simulink model "PhysicalArchitecture"  (R2020b)
settings: Solver=VariableStepAuto  StartTime=0.0  StopTime=10.0  RelTol=1e-3
model workspace (MAT data in the model file):
  DataToReport = Simulink.Bus
  DataToReport.Alignment = -1
  DataToReport.Elements_internal(1) = Simulink.BusElement
  DataToReport.Elements_internal(1).DimensionsMode = 'Fixed'
  DataToReport.Elements_internal(1).SamplingMode = 'Sample based'
  DataToReport.Elements_internal(1).SampleTime = -1
  DataToReport.Elements_internal(1).Name = 'Waypoints'
  DataToReport.Elements_internal(1).DataType_internal = 'double'
  DataToReport.Elements_internal(1).Complexity = 'real'
  DataToReport.Elements_internal(1).Dimensions = 1
  DataToReport.Elements_internal(2) = Simulink.BusElement
  DataToReport.Elements_internal(2).DimensionsMode = 'Fixed'
  DataToReport.Elements_internal(2).SamplingMode = 'Sample based'
  DataToReport.Elements_internal(2).SampleTime = -1
  DataToReport.Elements_internal(2).Name = 'VehicleLocation'
  DataToReport.Elements_internal(2).DataType_internal = 'double'
  DataToReport.Elements_internal(2).Complexity = 'real'
  DataToReport.Elements_internal(2).Dimensions = 1
  DataToReport.Elements_internal(3) = Simulink.BusElement
  DataToReport.Elements_internal(3).DimensionsMode = 'Fixed'
  DataToReport.Elements_internal(3).SamplingMode = 'Sample based'
  DataToReport.Elements_internal(3).SampleTime = -1
  DataToReport.Elements_internal(3).Name = 'TargetLocation'
  DataToReport.Elements_internal(3).DataType_internal = 'double'
  DataToReport.Elements_internal(3).Complexity = 'real'
  DataToReport.Elements_internal(3).Dimensions = 1
  DataToReport.Elements_internal(4) = Simulink.BusElement
  DataToReport.Elements_internal(4).DimensionsMode = 'Fixed'
  DataToReport.Elements_internal(4).SamplingMode = 'Sample based'
  DataToReport.Elements_internal(4).SampleTime = -1
  DataToReport.Elements_internal(4).Name = 'BatteryLevel'
  DataToReport.Elements_internal(4).DataType_internal = 'double'
  DataToReport.Elements_internal(4).Complexity = 'real'
  DataToReport.Elements_internal(4).Dimensions = 1
  DataToReport.DataScope = 'Auto'
settings Model: OrderedModelArguments=off  Creator=jantonio  LastModifiedBy=jantonio

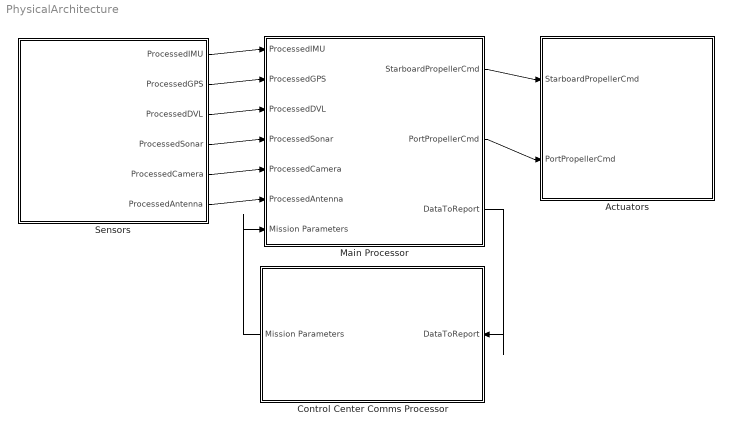
== system PhysicalArchitecture ==
  Actuators : Subsystem
      settings: PortSchema="{\"entries\":[{\"content\":{\"headerSize\":26,\"margin\":15,\"minimumSpacing\":25,\"sides\":[{\"content\":{\"connectorIds\":[\"In1\",\"In2\"]},\"type\":\"ConnectorPlacement.EquallySpacedRectSide\",\"uuid\":\"92d6a8cb-947e-47d6-81f8-e687db23cc48\"},{\"content\":{\"connectorIds\":[],\"side\":\"RIGHT\"},\"type\":\"ConnectorPlacement.EquallySpacedRectSide\",\"uuid\":\"2f71feb6-2a58-4436-853a-8f489ba40545\"},{\"content\":{\"connectorIds\":[],\"side\":\"TOP\"},\"type\":\"ConnectorPlacement.EquallySpacedRectSide\",\"uuid\":\"53be6a6a-df16-4e38-99d9-cb729dcfb7aa\"}]},\"type\":\"ConnectorPlacement.EquallySpacedConnector\",\"uuid\":\"6f13b966-c9d6-4990-a53d-58e940ab2e2e\"}],\"packageUris\":[\"http://schema.mathworks.com/mf0/Connector/19700101\"],\"version\":\"1.0\"}"
  Control Center Comms Processor : Subsystem
      settings: PortSchema="{\"entries\":[{\"content\":{\"headerSize\":26,\"margin\":15,\"minimumSpacing\":25,\"sides\":[{\"content\":{\"connectorIds\":[\"Out1\"]},\"type\":\"ConnectorPlacement.EquallySpacedRectSide\",\"uuid\":\"92d6a8cb-947e-47d6-81f8-e687db23cc48\"},{\"content\":{\"connectorIds\":[\"In1\"],\"side\":\"RIGHT\"},\"type\":\"ConnectorPlacement.EquallySpacedRectSide\",\"uuid\":\"2f71feb6-2a58-4436-853a-8f489ba40545\"},{\"content\":{\"connectorIds\":[],\"side\":\"TOP\"},\"type\":\"ConnectorPlacement.EquallySpacedRectSide\",\"uuid\":\"53be6a6a-df16-4e38-99d9-cb729dcfb7aa\"}]},\"type\":\"ConnectorPlacement.EquallySpacedConnector\",\"uuid\":\"6f13b966-c9d6-4990-a53d-58e940ab2e2e\"}],\"packageUris\":[\"http://schema.mathworks.com/mf0/Connector/19700101\"],\"version\":\"1.0\"}"
  Main Processor : Subsystem
      settings: PortSchema="{\"entries\":[{\"content\":{\"headerSize\":26,\"margin\":15,\"minimumSpacing\":25,\"sides\":[{\"content\":{\"connectorIds\":[\"In3\",\"In2\",\"In4\",\"In5\",\"In6\",\"In7\",\"In1\"]},\"type\":\"ConnectorPlacement.EquallySpacedRectSide\",\"uuid\":\"92d6a8cb-947e-47d6-81f8-e687db23cc48\"},{\"content\":{\"connectorIds\":[\"Out1\",\"Out2\",\"Out3\"],\"side\":\"RIGHT\"},\"type\":\"ConnectorPlacement.EquallySpacedRectSide\",\"uuid\":\"2f71feb6-2a58-4436-853a-8f489ba40545\"},{\"content\":{\"connectorIds\":[],\"side\":\"TOP\"},\"type\":\"ConnectorPlacement.EquallySpacedRectSide\",\"uuid\":\"53be6a6a-df16-4e38-99d9-cb729dcfb7aa\"},{\"content\":{\"connectorIds\":[],\"side\":\"BOTTOM\"},\"type\":\"ConnectorPlacement.EquallySpacedRectSide\",\"uuid\":\"d53c4466-3fe3-4f56-83bf-6f2fb5a5afe1\"}]},\"type\":\"ConnectorPlacement.EquallySpacedConnector\",\"uuid\":\"6f13b966-c9d6-4990-a53d-58e940ab2e2e\"}],\"packageUris\":[\"http://schema.mathworks.com/mf0/Connector/19700101\"],\"version\":\"1.0\"}"
  Sensors : Subsystem
      settings: PortSchema="{\"entries\":[{\"content\":{\"headerSize\":26,\"margin\":15,\"minimumSpacing\":25,\"sides\":[{\"content\":{\"connectorIds\":[]},\"type\":\"ConnectorPlacement.EquallySpacedRectSide\",\"uuid\":\"ebeba1ac-198c-4738-ae02-dee736f3e255\"},{\"content\":{\"connectorIds\":[\"Out1\",\"Out2\",\"Out3\",\"Out4\",\"Out6\",\"Out5\"],\"side\":\"RIGHT\"},\"type\":\"ConnectorPlacement.EquallySpacedRectSide\",\"uuid\":\"9a9b5092-10f1-44a7-a087-51aace0dbe34\"},{\"content\":{\"connectorIds\":[],\"side\":\"TOP\"},\"type\":\"ConnectorPlacement.EquallySpacedRectSide\",\"uuid\":\"96b74760-e30f-4e99-a3da-f77ce842a435\"}]},\"type\":\"ConnectorPlacement.EquallySpacedConnector\",\"uuid\":\"07af2d66-a99a-41b4-9a6d-4df096fe3f6b\"}],\"packageUris\":[\"http://schema.mathworks.com/mf0/Connector/19700101\"],\"version\":\"1.0\"}"
  wires:
  Sensors/1(ProcessedIMU) -> Main Processor/3(ProcessedIMU)
  Sensors/2(ProcessedGPS) -> Main Processor/2(ProcessedGPS)
  Sensors/5(ProcessedAntenna) -> Main Processor/7(ProcessedAntenna)
  Sensors/6(ProcessedCamera) -> Main Processor/6(ProcessedCamera)
  Sensors/4(ProcessedSonar) -> Main Processor/5(ProcessedSonar)
  Sensors/3(ProcessedDVL) -> Main Processor/4(ProcessedDVL)
  Main Processor/1(StarboardPropellerCmd) -> Actuators/1(StarboardPropellerCmd)
  Main Processor/2(PortPropellerCmd) -> Actuators/2(PortPropellerCmd)
  Control Center Comms Processor/1(Mission Parameters) -> Main Processor/1(Mission Parameters)
  Main Processor/3(DataToReport) -> Control Center Comms Processor/1(DataToReport)

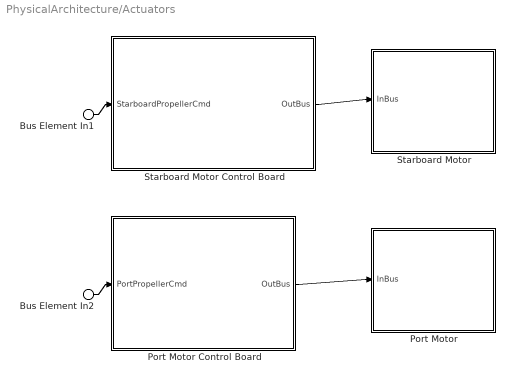
== system PhysicalArchitecture/Actuators ==
  Bus Element In1 : Inport  PortName=StarboardPropellerCmd
  Bus Element In2 : Inport  Port=2  PortName=PortPropellerCmd
  Port Motor : Subsystem
      settings: PortSchema="{\"entries\":[{\"content\":{\"headerSize\":26,\"margin\":15,\"minimumSpacing\":25,\"sides\":[{\"content\":{\"connectorIds\":[\"In1\"]},\"type\":\"ConnectorPlacement.EquallySpacedRectSide\",\"uuid\":\"92d6a8cb-947e-47d6-81f8-e687db23cc48\"},{\"content\":{\"connectorIds\":[],\"side\":\"RIGHT\"},\"type\":\"ConnectorPlacement.EquallySpacedRectSide\",\"uuid\":\"2f71feb6-2a58-4436-853a-8f489ba40545\"},{\"content\":{\"connectorIds\":[],\"side\":\"TOP\"},\"type\":\"ConnectorPlacement.EquallySpacedRectSide\",\"uuid\":\"53be6a6a-df16-4e38-99d9-cb729dcfb7aa\"}]},\"type\":\"ConnectorPlacement.EquallySpacedConnector\",\"uuid\":\"6f13b966-c9d6-4990-a53d-58e940ab2e2e\"}],\"packageUris\":[\"http://schema.mathworks.com/mf0/Connector/19700101\"],\"version\":\"1.0\"}"
  Port Motor Control Board : Subsystem
      settings: PortSchema="{\"entries\":[{\"content\":{\"headerSize\":26,\"margin\":15,\"minimumSpacing\":25,\"sides\":[{\"content\":{\"connectorIds\":[\"In1\"]},\"type\":\"ConnectorPlacement.EquallySpacedRectSide\",\"uuid\":\"92d6a8cb-947e-47d6-81f8-e687db23cc48\"},{\"content\":{\"connectorIds\":[\"Out1\"],\"side\":\"RIGHT\"},\"type\":\"ConnectorPlacement.EquallySpacedRectSide\",\"uuid\":\"2f71feb6-2a58-4436-853a-8f489ba40545\"},{\"content\":{\"connectorIds\":[],\"side\":\"TOP\"},\"type\":\"ConnectorPlacement.EquallySpacedRectSide\",\"uuid\":\"53be6a6a-df16-4e38-99d9-cb729dcfb7aa\"}]},\"type\":\"ConnectorPlacement.EquallySpacedConnector\",\"uuid\":\"6f13b966-c9d6-4990-a53d-58e940ab2e2e\"}],\"packageUris\":[\"http://schema.mathworks.com/mf0/Connector/19700101\"],\"version\":\"1.0\"}"
  Starboard Motor : Subsystem
      settings: PortSchema="{\"entries\":[{\"content\":{\"headerSize\":26,\"margin\":15,\"minimumSpacing\":25,\"sides\":[{\"content\":{\"connectorIds\":[\"In1\"]},\"type\":\"ConnectorPlacement.EquallySpacedRectSide\",\"uuid\":\"92d6a8cb-947e-47d6-81f8-e687db23cc48\"},{\"content\":{\"connectorIds\":[],\"side\":\"RIGHT\"},\"type\":\"ConnectorPlacement.EquallySpacedRectSide\",\"uuid\":\"2f71feb6-2a58-4436-853a-8f489ba40545\"},{\"content\":{\"connectorIds\":[],\"side\":\"TOP\"},\"type\":\"ConnectorPlacement.EquallySpacedRectSide\",\"uuid\":\"53be6a6a-df16-4e38-99d9-cb729dcfb7aa\"}]},\"type\":\"ConnectorPlacement.EquallySpacedConnector\",\"uuid\":\"6f13b966-c9d6-4990-a53d-58e940ab2e2e\"}],\"packageUris\":[\"http://schema.mathworks.com/mf0/Connector/19700101\"],\"version\":\"1.0\"}"
  Starboard Motor Control Board : Subsystem
      settings: PortSchema="{\"entries\":[{\"content\":{\"headerSize\":26,\"margin\":15,\"minimumSpacing\":25,\"sides\":[{\"content\":{\"connectorIds\":[\"In1\"]},\"type\":\"ConnectorPlacement.EquallySpacedRectSide\",\"uuid\":\"92d6a8cb-947e-47d6-81f8-e687db23cc48\"},{\"content\":{\"connectorIds\":[\"Out1\"],\"side\":\"RIGHT\"},\"type\":\"ConnectorPlacement.EquallySpacedRectSide\",\"uuid\":\"2f71feb6-2a58-4436-853a-8f489ba40545\"},{\"content\":{\"connectorIds\":[],\"side\":\"TOP\"},\"type\":\"ConnectorPlacement.EquallySpacedRectSide\",\"uuid\":\"53be6a6a-df16-4e38-99d9-cb729dcfb7aa\"}]},\"type\":\"ConnectorPlacement.EquallySpacedConnector\",\"uuid\":\"6f13b966-c9d6-4990-a53d-58e940ab2e2e\"}],\"packageUris\":[\"http://schema.mathworks.com/mf0/Connector/19700101\"],\"version\":\"1.0\"}"
  wires:
  Starboard Motor Control Board/1(OutBus) -> Starboard Motor/1(InBus)
  Port Motor Control Board/1(OutBus) -> Port Motor/1(InBus)
  Bus Element In1/1 -> Starboard Motor Control Board/1(StarboardPropellerCmd)
  Bus Element In2/1 -> Port Motor Control Board/1(PortPropellerCmd)

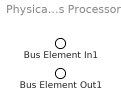
== system PhysicalArchitecture/Control Center Comms Processor ==
  Bus Element In1 : Inport  PortName=DataToReport
  Bus Element Out1 : Outport  PortName=Mission Parameters

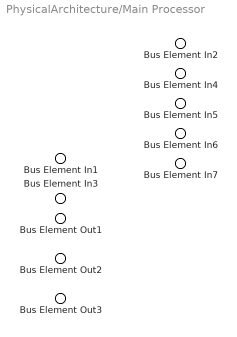
== system PhysicalArchitecture/Main Processor ==
  Bus Element In7 : Inport  PortName=Mission Parameters
  Bus Element In2 : Inport  Port=2  PortName=ProcessedGPS
  Bus Element In1 : Inport  Port=3  PortName=ProcessedIMU
  Bus Element In6 : Inport  Port=4  PortName=ProcessedDVL
  Bus Element In5 : Inport  Port=5  PortName=ProcessedSonar
  Bus Element In4 : Inport  Port=6  PortName=ProcessedCamera
  Bus Element In3 : Inport  Port=7  PortName=ProcessedAntenna
  Bus Element Out1 : Outport  PortName=StarboardPropellerCmd
  Bus Element Out2 : Outport  Port=2  PortName=PortPropellerCmd
  Bus Element Out3 : Outport  Port=3  PortName=DataToReport

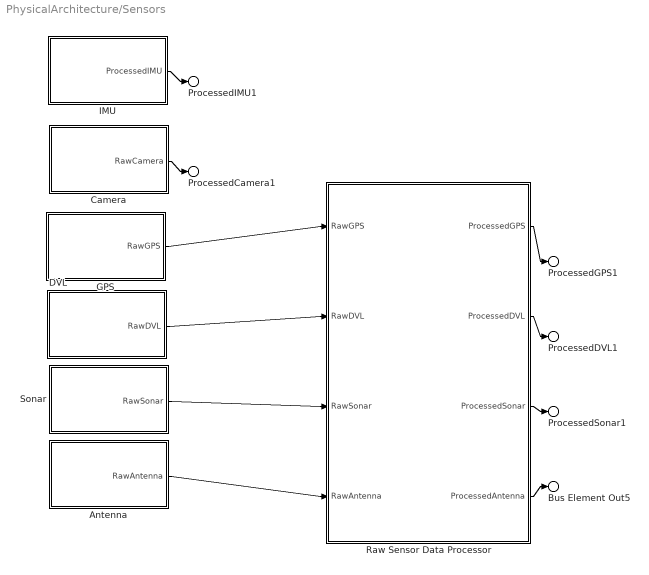
== system PhysicalArchitecture/Sensors ==
  Antenna : Subsystem
      settings: PortSchema="{\"entries\":[{\"content\":{\"headerSize\":26,\"margin\":15,\"minimumSpacing\":25,\"sides\":[{\"content\":{\"connectorIds\":[]},\"type\":\"ConnectorPlacement.EquallySpacedRectSide\",\"uuid\":\"39ab5f6e-200b-418c-957c-0427e0a2d192\"},{\"content\":{\"connectorIds\":[\"Out1\"],\"side\":\"RIGHT\"},\"type\":\"ConnectorPlacement.EquallySpacedRectSide\",\"uuid\":\"2abcd6b7-9ef0-4689-b904-6f1a8a48cdb7\"},{\"content\":{\"connectorIds\":[],\"side\":\"TOP\"},\"type\":\"ConnectorPlacement.EquallySpacedRectSide\",\"uuid\":\"3ddcf8bd-fb65-4c69-ae6b-4c30928b7beb\"}]},\"type\":\"ConnectorPlacement.EquallySpacedConnector\",\"uuid\":\"ab0c7103-d8ef-4055-8653-3cf105b5edbd\"}],\"packageUris\":[\"http://schema.mathworks.com/mf0/Connector/19700101\"],\"version\":\"1.0\"}"
  Camera : Subsystem
      settings: PortSchema="{\"entries\":[{\"content\":{\"headerSize\":26,\"margin\":15,\"minimumSpacing\":25,\"sides\":[{\"content\":{\"connectorIds\":[]},\"type\":\"ConnectorPlacement.EquallySpacedRectSide\",\"uuid\":\"39ab5f6e-200b-418c-957c-0427e0a2d192\"},{\"content\":{\"connectorIds\":[\"Out1\"],\"side\":\"RIGHT\"},\"type\":\"ConnectorPlacement.EquallySpacedRectSide\",\"uuid\":\"2abcd6b7-9ef0-4689-b904-6f1a8a48cdb7\"},{\"content\":{\"connectorIds\":[],\"side\":\"TOP\"},\"type\":\"ConnectorPlacement.EquallySpacedRectSide\",\"uuid\":\"3ddcf8bd-fb65-4c69-ae6b-4c30928b7beb\"}]},\"type\":\"ConnectorPlacement.EquallySpacedConnector\",\"uuid\":\"ab0c7103-d8ef-4055-8653-3cf105b5edbd\"}],\"packageUris\":[\"http://schema.mathworks.com/mf0/Connector/19700101\"],\"version\":\"1.0\"}"
  DVL : Subsystem
      settings: PortSchema="{\"entries\":[{\"content\":{\"headerSize\":26,\"margin\":15,\"minimumSpacing\":25,\"sides\":[{\"content\":{\"connectorIds\":[]},\"type\":\"ConnectorPlacement.EquallySpacedRectSide\",\"uuid\":\"39ab5f6e-200b-418c-957c-0427e0a2d192\"},{\"content\":{\"connectorIds\":[\"Out1\"],\"side\":\"RIGHT\"},\"type\":\"ConnectorPlacement.EquallySpacedRectSide\",\"uuid\":\"2abcd6b7-9ef0-4689-b904-6f1a8a48cdb7\"},{\"content\":{\"connectorIds\":[],\"side\":\"TOP\"},\"type\":\"ConnectorPlacement.EquallySpacedRectSide\",\"uuid\":\"3ddcf8bd-fb65-4c69-ae6b-4c30928b7beb\"}]},\"type\":\"ConnectorPlacement.EquallySpacedConnector\",\"uuid\":\"ab0c7103-d8ef-4055-8653-3cf105b5edbd\"}],\"packageUris\":[\"http://schema.mathworks.com/mf0/Connector/19700101\"],\"version\":\"1.0\"}"
  GPS : Subsystem
      settings: PortSchema="{\"entries\":[{\"content\":{\"headerSize\":26,\"margin\":15,\"minimumSpacing\":25,\"sides\":[{\"content\":{\"connectorIds\":[]},\"type\":\"ConnectorPlacement.EquallySpacedRectSide\",\"uuid\":\"39ab5f6e-200b-418c-957c-0427e0a2d192\"},{\"content\":{\"connectorIds\":[\"Out1\"],\"side\":\"RIGHT\"},\"type\":\"ConnectorPlacement.EquallySpacedRectSide\",\"uuid\":\"2abcd6b7-9ef0-4689-b904-6f1a8a48cdb7\"},{\"content\":{\"connectorIds\":[],\"side\":\"TOP\"},\"type\":\"ConnectorPlacement.EquallySpacedRectSide\",\"uuid\":\"3ddcf8bd-fb65-4c69-ae6b-4c30928b7beb\"}]},\"type\":\"ConnectorPlacement.EquallySpacedConnector\",\"uuid\":\"ab0c7103-d8ef-4055-8653-3cf105b5edbd\"}],\"packageUris\":[\"http://schema.mathworks.com/mf0/Connector/19700101\"],\"version\":\"1.0\"}"
  IMU : Subsystem
      settings: PortSchema="{\"entries\":[{\"content\":{\"headerSize\":26,\"margin\":15,\"minimumSpacing\":25,\"sides\":[{\"content\":{\"connectorIds\":[]},\"type\":\"ConnectorPlacement.EquallySpacedRectSide\",\"uuid\":\"39ab5f6e-200b-418c-957c-0427e0a2d192\"},{\"content\":{\"connectorIds\":[\"Out1\"],\"side\":\"RIGHT\"},\"type\":\"ConnectorPlacement.EquallySpacedRectSide\",\"uuid\":\"2abcd6b7-9ef0-4689-b904-6f1a8a48cdb7\"},{\"content\":{\"connectorIds\":[],\"side\":\"TOP\"},\"type\":\"ConnectorPlacement.EquallySpacedRectSide\",\"uuid\":\"3ddcf8bd-fb65-4c69-ae6b-4c30928b7beb\"}]},\"type\":\"ConnectorPlacement.EquallySpacedConnector\",\"uuid\":\"ab0c7103-d8ef-4055-8653-3cf105b5edbd\"}],\"packageUris\":[\"http://schema.mathworks.com/mf0/Connector/19700101\"],\"version\":\"1.0\"}"
  Raw Sensor Data Processor : Subsystem
      settings: PortSchema="{\"entries\":[{\"content\":{\"headerSize\":26,\"margin\":15,\"minimumSpacing\":25,\"sides\":[{\"content\":{\"connectorIds\":[\"In1\",\"In2\",\"In3\",\"In4\"]},\"type\":\"ConnectorPlacement.EquallySpacedRectSide\",\"uuid\":\"92d6a8cb-947e-47d6-81f8-e687db23cc48\"},{\"content\":{\"connectorIds\":[\"Out1\",\"Out2\",\"Out3\",\"Out4\"],\"side\":\"RIGHT\"},\"type\":\"ConnectorPlacement.EquallySpacedRectSide\",\"uuid\":\"2f71feb6-2a58-4436-853a-8f489ba40545\"},{\"content\":{\"connectorIds\":[],\"side\":\"TOP\"},\"type\":\"ConnectorPlacement.EquallySpacedRectSide\",\"uuid\":\"53be6a6a-df16-4e38-99d9-cb729dcfb7aa\"}]},\"type\":\"ConnectorPlacement.EquallySpacedConnector\",\"uuid\":\"6f13b966-c9d6-4990-a53d-58e940ab2e2e\"}],\"packageUris\":[\"http://schema.mathworks.com/mf0/Connector/19700101\"],\"version\":\"1.0\"}"
  Sonar : Subsystem
      settings: PortSchema="{\"entries\":[{\"content\":{\"headerSize\":26,\"margin\":15,\"minimumSpacing\":25,\"sides\":[{\"content\":{\"connectorIds\":[]},\"type\":\"ConnectorPlacement.EquallySpacedRectSide\",\"uuid\":\"39ab5f6e-200b-418c-957c-0427e0a2d192\"},{\"content\":{\"connectorIds\":[\"Out1\"],\"side\":\"RIGHT\"},\"type\":\"ConnectorPlacement.EquallySpacedRectSide\",\"uuid\":\"2abcd6b7-9ef0-4689-b904-6f1a8a48cdb7\"},{\"content\":{\"connectorIds\":[],\"side\":\"TOP\"},\"type\":\"ConnectorPlacement.EquallySpacedRectSide\",\"uuid\":\"3ddcf8bd-fb65-4c69-ae6b-4c30928b7beb\"}]},\"type\":\"ConnectorPlacement.EquallySpacedConnector\",\"uuid\":\"ab0c7103-d8ef-4055-8653-3cf105b5edbd\"}],\"packageUris\":[\"http://schema.mathworks.com/mf0/Connector/19700101\"],\"version\":\"1.0\"}"
  ProcessedIMU1 : Outport  PortName=ProcessedIMU
  ProcessedGPS1 : Outport  Port=2  PortName=ProcessedGPS
  ProcessedDVL1 : Outport  Port=3  PortName=ProcessedDVL
  ProcessedSonar1 : Outport  Port=4  PortName=ProcessedSonar
  Bus Element Out5 : Outport  Port=5  PortName=ProcessedAntenna
  ProcessedCamera1 : Outport  Port=6  PortName=ProcessedCamera
  wires:
  IMU/1(ProcessedIMU) -> ProcessedIMU1/1
  Camera/1(RawCamera) -> ProcessedCamera1/1
  GPS/1(RawGPS) -> Raw Sensor Data Processor/1(RawGPS)
  DVL/1(RawDVL) -> Raw Sensor Data Processor/2(RawDVL)
  Sonar/1(RawSonar) -> Raw Sensor Data Processor/3(RawSonar)
  Antenna/1(RawAntenna) -> Raw Sensor Data Processor/4(RawAntenna)
  Raw Sensor Data Processor/1(ProcessedGPS) -> ProcessedGPS1/1
  Raw Sensor Data Processor/2(ProcessedDVL) -> ProcessedDVL1/1
  Raw Sensor Data Processor/3(ProcessedSonar) -> ProcessedSonar1/1
  Raw Sensor Data Processor/4(ProcessedAntenna) -> Bus Element Out5/1

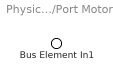
== system PhysicalArchitecture/Actuators/Port Motor ==
  Bus Element In1 : Inport  PortName=InBus

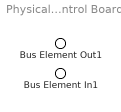
== system PhysicalArchitecture/Actuators/Port Motor Control Board ==
  Bus Element In1 : Inport  PortName=PortPropellerCmd
  Bus Element Out1 : Outport  PortName=OutBus

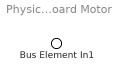
== system PhysicalArchitecture/Actuators/Starboard Motor ==
  Bus Element In1 : Inport  PortName=InBus

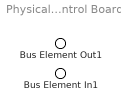
== system PhysicalArchitecture/Actuators/Starboard Motor Control Board ==
  Bus Element In1 : Inport  PortName=StarboardPropellerCmd
  Bus Element Out1 : Outport  PortName=OutBus

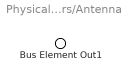
== system PhysicalArchitecture/Sensors/Antenna ==
  Bus Element Out1 : Outport  PortName=RawAntenna

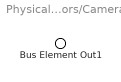
== system PhysicalArchitecture/Sensors/Camera ==
  Bus Element Out1 : Outport  PortName=RawCamera

== system PhysicalArchitecture/Sensors/DVL ==
  Bus Element Out1 : Outport  PortName=RawDVL

== system PhysicalArchitecture/Sensors/GPS ==
  Bus Element Out1 : Outport  PortName=RawGPS

== system PhysicalArchitecture/Sensors/IMU ==
  Bus Element Out1 : Outport  PortName=ProcessedIMU

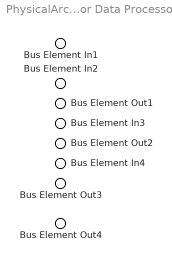
== system PhysicalArchitecture/Sensors/Raw Sensor Data Processor ==
  Bus Element In1 : Inport  PortName=RawGPS
  Bus Element In2 : Inport  Port=2  PortName=RawDVL
  Bus Element In3 : Inport  Port=3  PortName=RawSonar
  Bus Element In4 : Inport  Port=4  PortName=RawAntenna
  Bus Element Out1 : Outport  PortName=ProcessedGPS
  Bus Element Out2 : Outport  Port=2  PortName=ProcessedDVL
  Bus Element Out3 : Outport  Port=3  PortName=ProcessedSonar
  Bus Element Out4 : Outport  Port=4  PortName=ProcessedAntenna

== system PhysicalArchitecture/Sensors/Sonar ==
  Bus Element Out1 : Outport  PortName=RawSonar
